simulink model "half"  (R2019b)
settings: Solver=VariableStepAuto  StartTime=0.0  StopTime=10.0  RelTol=1e-5
values from neighbouring files (symbols this model uses):
  A_1 = [0 0 1 0 ... (first row only)    [main.m]
  A_2 = [0 1 ... (first row only)    [main.m]
  B_1 = [0 0 ... (first row only)    [main.m]
  B_2 = [0 0 ... (first row only)    [main.m]
  R = 0.05    [main.m]
undefined symbols (not defined in the file or in its folder): K_1, K_2
libraries: simulink x2
settings Model: Creator=Jamie  LastModifiedBy=Jamie
settings SolverCC: MaxConsecutiveZCs=100  MaxConsecutiveMinStep=100

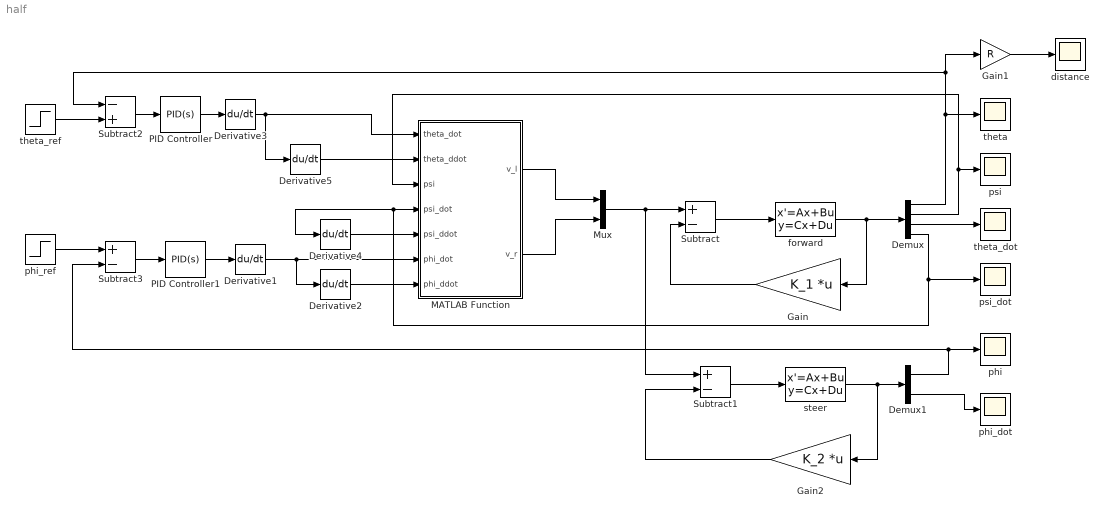
== system half ==
  Demux : Demux
  Demux1 : Demux  Outputs=2
  Derivative{1..5} (5 alike) : Derivative
  Gain : Gain  Gain=K_1  Multiplication=Matrix(K*u)
  Gain1 : Gain  Gain=R
  Gain2 : Gain  Gain=K_2  Multiplication=Matrix(K*u)
  MATLAB Function : MATLAB Function  TreatAsAtomicUnit=on
  Mux : Mux  Inputs=2
  PID Controller : simulink/Continuous/PID Controller  Controller=PID  Form=Parallel  TimeDomain=Continuous-time  SampleTime=-1  IntegratorMethod=Forward Euler  FilterMethod=Forward Euler  ControllerParametersSource=internal  P=1000  I=1  D=100  UseFilter=on  N=100  TunerSelectOption=Transfer Function Based (PID Tuner App)  InitialConditionSource=internal  InitialConditionForIntegrator=0  InitialConditionForFilter=0  DifferentiatorICPrevScaledInput=0  ExternalReset=none  TrackingMode=off  Kt=1  LimitOutput=off  UpperSaturationLimit=inf  LowerSaturationLimit=-inf  LinearizeAsGain=on  AntiWindupMode=none  Kb=1  POutMin=[]  POutMax=[]  IOutMin=[]  IOutMax=[]  DOutMin=[]  DOutMax=[]  NOutMin=[]  NOutMax=[]  SumOutMin=[]  SumOutMax=[]  SaturationOutMin=[]  SaturationOutMax=[]  PParamMin=[]  PParamMax=[]  IParamMin=[]  IParamMax=[]  DParamMin=[]  DParamMax=[]  NParamMin=[]  NParamMax=[]  KbParamMin=[]  KbParamMax=[]  KtParamMin=[]  KtParamMax=[]  KbOutMin=[]  KbOutMax=[]  KtOutMin=[]  KtOutMax=[]  IntegratorOutMin=[]  IntegratorOutMax=[]  FilterOutMin=[]  FilterOutMax=[]  SumI1OutMin=[]  SumI1OutMax=[]  SumI2OutMin=[]  SumI2OutMax=[]  SumI3OutMin=[]  SumI3OutMax=[]  SumI4OutMin=[]  SumI4OutMax=[]  SumDOutMin=[]  SumDOutMax=[]  DifferentiatorOutMin=[]  DifferentiatorOutMax=[]  FilterDiffOutCoefMin=[]  FilterDiffOutCoefMax=[]  ReciprocalOutMin=[]  ReciprocalOutMax=[]  SumDenOutMin=[]  SumDenOutMax=[]  SumNumOutMin=[]  SumNumOutMax=[]  DivideOutMin=[]  DivideOutMax=[]  IntegratorContinuousStateAttributes=''  IntegratorStateMustResolveToSignalObject=off  IntegratorRTWStateStorageClass=Auto  FilterContinuousStateAttributes=''  FilterStateMustResolveToSignalObject=off  FilterRTWStateStorageClass=Auto  ParallelPVariant=InternalParameters  IdealPVariant=Disabled  IVariant=InternalParameters  DVariant=InternalParameters  IntegratorVariant=Continuous  SatVariant=Disabled  AWVariant=Passthrough  PCopyVariant=Disabled  TRVariant=Disabled  FdbkBlocksVariant=Forward  IdealPFdbkVariant=Disabled  SatFdbkVariant=Disabled  DerivativeFilterVariant=ContFilter  NVariant=InternalParameters  NCopyVariant=Disabled  FilterICVariant=InternalICsFilter  IntegratorICVariant=InternalICs  ExternalResetVariant=Disabled  TRSumVariant=Passthrough  SumFdbkVariant=Disabled  SumVariant=Sum_PID
  PID Controller1 : simulink/Continuous/PID Controller  Controller=PID  Form=Parallel  TimeDomain=Continuous-time  SampleTime=-1  IntegratorMethod=Forward Euler  FilterMethod=Forward Euler  ControllerParametersSource=internal  P=1000  I=1  D=100  UseFilter=on  N=100  TunerSelectOption=Transfer Function Based (PID Tuner App)  InitialConditionSource=internal  InitialConditionForIntegrator=0  InitialConditionForFilter=0  DifferentiatorICPrevScaledInput=0  ExternalReset=none  TrackingMode=off  Kt=1  LimitOutput=off  UpperSaturationLimit=inf  LowerSaturationLimit=-inf  LinearizeAsGain=on  AntiWindupMode=none  Kb=1  POutMin=[]  POutMax=[]  IOutMin=[]  IOutMax=[]  DOutMin=[]  DOutMax=[]  NOutMin=[]  NOutMax=[]  SumOutMin=[]  SumOutMax=[]  SaturationOutMin=[]  SaturationOutMax=[]  PParamMin=[]  PParamMax=[]  IParamMin=[]  IParamMax=[]  DParamMin=[]  DParamMax=[]  NParamMin=[]  NParamMax=[]  KbParamMin=[]  KbParamMax=[]  KtParamMin=[]  KtParamMax=[]  KbOutMin=[]  KbOutMax=[]  KtOutMin=[]  KtOutMax=[]  IntegratorOutMin=[]  IntegratorOutMax=[]  FilterOutMin=[]  FilterOutMax=[]  SumI1OutMin=[]  SumI1OutMax=[]  SumI2OutMin=[]  SumI2OutMax=[]  SumI3OutMin=[]  SumI3OutMax=[]  SumI4OutMin=[]  SumI4OutMax=[]  SumDOutMin=[]  SumDOutMax=[]  DifferentiatorOutMin=[]  DifferentiatorOutMax=[]  FilterDiffOutCoefMin=[]  FilterDiffOutCoefMax=[]  ReciprocalOutMin=[]  ReciprocalOutMax=[]  SumDenOutMin=[]  SumDenOutMax=[]  SumNumOutMin=[]  SumNumOutMax=[]  DivideOutMin=[]  DivideOutMax=[]  IntegratorContinuousStateAttributes=''  IntegratorStateMustResolveToSignalObject=off  IntegratorRTWStateStorageClass=Auto  FilterContinuousStateAttributes=''  FilterStateMustResolveToSignalObject=off  FilterRTWStateStorageClass=Auto  ParallelPVariant=InternalParameters  IdealPVariant=Disabled  IVariant=InternalParameters  DVariant=InternalParameters  IntegratorVariant=Continuous  SatVariant=Disabled  AWVariant=Passthrough  PCopyVariant=Disabled  TRVariant=Disabled  FdbkBlocksVariant=Forward  IdealPFdbkVariant=Disabled  SatFdbkVariant=Disabled  DerivativeFilterVariant=ContFilter  NVariant=InternalParameters  NCopyVariant=Disabled  FilterICVariant=InternalICsFilter  IntegratorICVariant=InternalICs  ExternalResetVariant=Disabled  TRSumVariant=Passthrough  SumFdbkVariant=Disabled  SumVariant=Sum_PID
  Subtract : Sum  Inputs=+-
  Subtract1 : Sum  Inputs=+-
  Subtract2 : Sum  Inputs=-+
  Subtract3 : Sum  Inputs=+-
  distance : Scope
  forward : StateSpace  A=A_1  B=B_1  C=[1 0 0 0; 0 1 0 0; 0 0 0 0; 0 0 0 0]  D=[0 0; 0 0; 0 0; 0 0]  InitialCondition=0
  phi : Scope
  phi_dot : Scope
  phi_ref : Step  After=0.5  SampleTime=0
  psi : Scope
  psi_dot : Scope
  steer : StateSpace  A=A_2  B=B_2  C=eye(2)  D=[0 0; 0 0]  InitialCondition=0
  theta : Scope
  theta_dot : Scope
  theta_ref : Step  SampleTime=0
  wires:
  MATLAB Function/2(v_r) -> Mux/2
  MATLAB Function/1(v_l) -> Mux/1
  forward/1 -> Demux/1, Gain/1
  steer/1 -> Demux1/1, Gain2/1
  Demux1/1 -> phi/1, Subtract3/2
  Demux1/2 -> phi_dot/1
  Demux/1 -> Subtract2/1, Gain1/1, theta/1
  Demux/2 -> MATLAB Function/3(psi), psi/1
  Demux/4 -> MATLAB Function/4(psi_dot), Derivative4/1, psi_dot/1
  Subtract/1 -> forward/1
  Mux/1 -> Subtract1/1, Subtract/1
  Gain2/1 -> Subtract1/2
  Subtract1/1 -> steer/1
  Gain/1 -> Subtract/2
  Gain1/1 -> distance/1
  Subtract3/1 -> PID Controller1/1
  Subtract2/1 -> PID Controller/1
  PID Controller1/1 -> Derivative1/1
  Derivative1/1 -> Derivative2/1, MATLAB Function/6(phi_dot)
  Derivative2/1 -> MATLAB Function/7(phi_ddot)
  Derivative4/1 -> MATLAB Function/5(psi_ddot)
  PID Controller/1 -> Derivative3/1
  Derivative5/1 -> MATLAB Function/2(theta_ddot)
  Derivative3/1 -> MATLAB Function/1(theta_dot), Derivative5/1
  Demux/3 -> theta_dot/1
  theta_ref/1 -> Subtract2/2
  phi_ref/1 -> Subtract3/1

== matlab function half/MATLAB Function ==
  data: theta_dot input; theta_ddot input; psi input; psi_dot input; v_l output; psi_ddot input; phi_dot input; phi_ddot input; v_r output
function [v_l, v_r] = fcn(theta_dot, theta_ddot, psi, psi_dot, psi_ddot, phi_dot, phi_ddot)
%system specification error parameter
p_ss = 1.05;

m = 0.08;
R = 0.05;
M = 0.77;
W = 0.12;
H = 0.16;
D = 0.04;

L = H/2;
J_w = (m*R^2)/2;
J_phi = M*(W^2 + D^2)/12;
J_m = 1e-5;
R_m = 6.69;
K_b = 0.47;
K_t = 0.32;
n = 1;
f_m = 0.0022;
f_w = 0;

m_ss = m*p_ss;
R_ss = R*p_ss;
M_ss = M*p_ss;
W_ss = W*p_ss;

theta_l_dot = theta_dot - W_ss*phi_dot/(2*R_ss);
theta_r_dot = theta_dot + W_ss*phi_dot/(2*R_ss);

% if theta_ddot > 100
%     theta_ddot = 100;
% elseif theta_ddot < -100
%     theta_ddot = -100;
% end
    
F_theta = ((2*m_ss + M_ss)*R_ss^2 + 2*J_w + 2*n^2*J_m)*theta_ddot + (M_ss*L*R_ss*cos(psi) - 2*n^2*J_m)*psi_ddot - M_ss*L*R_ss*psi_dot^2*sin(psi);
% F_psi = (M_ss*L*R_ss*cos(psi) - 2*n^2*J_m)*theta_ddot + (M_ss*L^2 + J_psi + 2*n^2*J_m)*psi_ddot - M_ss*g*L*sin(psi) - M_ss*L^2*phi_dot^2*sin(psi)*cos(psi);
F_phi = (m_ss*W_ss^2/2 + J_phi + W_ss^2/(2*R_ss^2)*(J_w + n^2*J_m) + M_ss*L^2*(sin(psi))^2)*phi_ddot + 2*M_ss*L^2*psi_dot*phi_dot*sin(psi)*cos(psi);

F_l = F_theta/2 - R_ss*F_phi/W_ss;
F_r = F_theta/2 + R_ss*F_phi/W_ss;

i_l = (F_l + f_w*theta_l_dot - f_m*(psi_dot - theta_l_dot))/(n*K_t); 
i_r = (F_r + f_w*theta_r_dot - f_m*(psi_dot - theta_r_dot))/(n*K_t); 

v_l = i_l*R_m - K_b*(psi_dot - theta_l_dot);  
v_r = i_r*R_m - K_b*(psi_dot - theta_r_dot);
